simulink subsystem "Disable_Gains"  (R2023a)
settings: Solver=VariableStepAuto  StartTime=0.0  StopTime=10.0  RelTol=1e-3

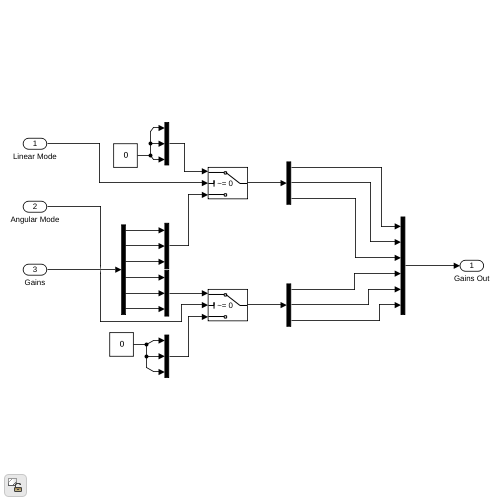
[thumbnail: Simulink's stored preview of the top-level diagram]
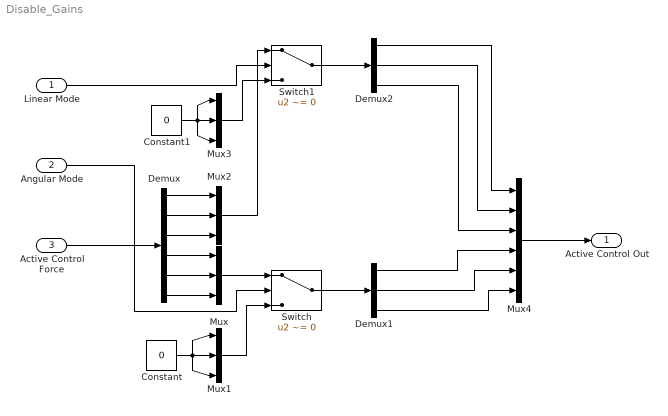
== system Disable_Gains ==
  Linear Mode : Inport
  Angular Mode : Inport  Port=2
  Active Control Force : Inport  Port=3
  Constant : Constant  Value=0
  Constant1 : Constant  Value=0
  Demux : Demux  Outputs=6
  Demux1 : Demux  Outputs=3
  Demux2 : Demux  Outputs=3
  Mux{,1..3} (4 alike) : Mux  Inputs=3
  Mux4 : Mux  Inputs=6
  Switch : Switch  Criteria=u2 ~= 0  SaturateOnIntegerOverflow=off  InputSameDT=off
  Switch1 : Switch  Criteria=u2 ~= 0  SaturateOnIntegerOverflow=off  InputSameDT=off
  Active Control Out : Outport
  wires:
  Active Control Force/1 -> Demux/1
  Demux/4 -> Mux/1
  Demux/5 -> Mux/2
  Demux/6 -> Mux/3
  Mux/1 -> Switch/1
  Angular Mode/1 -> Switch/2
  Constant/1 -> Mux1/2, Mux1/3, Mux1/1
  Mux1/1 -> Switch/3
  Switch/1 -> Demux1/1
  Demux/1 -> Mux2/1
  Demux/2 -> Mux2/2
  Demux/3 -> Mux2/3
  Mux2/1 -> Switch1/1
  Constant1/1 -> Mux3/2, Mux3/3, Mux3/1
  Linear Mode/1 -> Switch1/2
  Switch1/1 -> Demux2/1
  Demux1/1 -> Mux4/4
  Demux1/2 -> Mux4/5
  Demux1/3 -> Mux4/6
  Demux2/3 -> Mux4/3
  Demux2/2 -> Mux4/2
  Demux2/1 -> Mux4/1
  Mux4/1 -> Active Control Out/1
  Mux3/1 -> Switch1/3
